simulink model "Boeing787_Yue"  (R2013a)
settings: Solver=ode23tb  SolverMode=SingleTasking  StartTime=0.0  StopTime=346  RelTol=1e-3
InitFcn:
  | load('SampleOutput.mat')
  | 
  | load('SampleFuelBurn.mat')
values from neighbouring files (symbols this model uses):
  FuelBurn = [0 0 0 0 0 0 0 0 0 0 0 0 ... (18249 elements, 1x18249)]    [Benchmark_data1.mat]
undefined symbols (not defined in the file or in its folder): ailerons, AirProp, B_737, elevator, HydProp, landing_gear, rudder, thrust_rev
libraries: PowerFlowLib x118, simulink x20
(part 18 of 26)

== system Boeing787_Yue/Electrical/Generation Unit Sync-Sync6 ==
  engine speed : Inport
  idq0 : Inport  Port=2
  Temperature : Inport  Port=3
  Bus Creator : BusCreator  Inputs=3
  Bus Creator1 : BusCreator  Inputs=3
  Coeff of Resistance : Gain  Gain=3.85e-3
  Demux : Demux  Outputs=3
  Gain : Gain  Gain=200*2/3
  Gain1 : Gain  Gain=200
  Generator : Subsystem
      mask Display:
      | p = 0:0.1:(2*pi+0.1);
      | plot(sin(p), cos(p));
      | p1 = (-pi/8-0.1-0.2):0.1:(pi/8+0.1-0.2);
      | plot(0.8*sin(p1), 0.8*cos(p1), 0.8*sin(p1+pi), 0.8*cos(p1+pi));
      | p2 = sin((-pi/8-0.1-0.2+pi/8+0.1-0.2)/2);
      | p3 = sin((-pi/8-0.1-0.2+pi/8+0.1-0.2)/2+pi);
      | p4 = cos((-pi/8-0.1-0.2+pi/8+0.1-0.2)/2);
      | p5 = cos((-pi/8-0.1-0.2+pi/8+0.1-0.2)/2+pi);
      | plot(0.8*[p2, p3], 0.8*[p4, p5]);
      | port_label('output', 1, 'Vdq0');
      | port_label('output', 2, 'Te');
      | port_label('output', 3, 'Vfd');
      | port_label('output', 4, 'Ploss');
      | port_label('input', 1, 'idq0');
      | port_label('input', 2, 'w');
      | port_label('input', 3, 'ifd');
  Initial Temperature : Constant  Value=25
  Memory : Memory
  Permanent Magnet Synchronous Generator1 : PowerFlowLib/Energy & Power Systems/Electrical/Machines/Permanent Magnet Synchronous Generator1
  RPM_to_radps : Gain  Gain=pi/30
  Scope2 : Scope
      settings: TimeRange=100  YMin=0  YMax=5500
  Sum : Sum  Inputs=++|
  Sum1 : Sum
  Sum5 : Sum  Inputs=|+-
  Sum6 : Sum  Inputs=|++
  control1 : Constant
  data_sink : PowerFlowLib/Support Functions//Tools/data_sink
  one : Constant
  three-phase active rectifier Voltage Mode : PowerFlowLib/Energy & Power Systems/Electrical/Rectifiers/three-phase  active rectifier Voltage Mode  L=1  C=1e-4
  vdq0 : Outport
  engine torque : Outport  Port=2
  Ploss : Outport  Port=3
  wires:
  [R_temp_delta] -> Generator/4(Temp)
  engine speed/1 -> RPM_to_radps/1
  Bus Creator1/1 -> Bus Creator/1  "vdq0 (V)"
  Demux/3 -> Bus Creator1/3  "v0"
  Demux/2 -> Bus Creator1/2  "vq"
  Demux/1 -> Bus Creator1/1  "vd"
  Bus Creator/1 -> data_sink/1
  Sum/1 -> engine torque/1
  RPM_to_radps/1 -> Scope2/1, Generator/2(w), Permanent Magnet Synchronous Generator1/2
  Permanent Magnet Synchronous Generator1/1 -> three-phase active rectifier Voltage Mode/1
  control1/1 -> three-phase active rectifier Voltage Mode/2
  Generator/3(vfd') -> Gain1/1
  Gain1/1 -> three-phase active rectifier Voltage Mode/3
  Gain/1 -> Generator/3(ifd'), Bus Creator/3  "Excit current (A)"
  three-phase active rectifier Voltage Mode/1 -> Gain/1
  three-phase active rectifier Voltage Mode/2 -> Memory/1
  Permanent Magnet Synchronous Generator1/2 -> Sum/1
  Generator/2(Te) -> Sum/2
  Generator/1(vdq0) -> Demux/1, vdq0/1  "Vdq0 (V)"
  Permanent Magnet Synchronous Generator1/3 -> Sum1/1
  Generator/4(Ploss) -> Sum1/2
  Sum1/1 -> Bus Creator/2, Ploss/1  "Ploss (W)"
  Memory/1 -> Permanent Magnet Synchronous Generator1/1
  Sum6/1 -> [R_temp_delta]
  one/1 -> Sum6/2
  Coeff of Resistance/1 -> Sum6/1
  Sum5/1 -> Coeff of Resistance/1
  Initial Temperature/1 -> Sum5/2
  Temperature/1 -> Sum5/1
  idq0/1 -> Generator/1(idq0)

== system Boeing787_Yue/Electrical/Loads ==
  Constant : Constant  Value=[150,0,0]
  Constant1 : Constant  Value=[150 0 0]
  Constant2 : Constant  Value=[150 0]
  Constant3 : Constant  Value=[150 0]
  ElectricalSource1 : PowerFlowLib/Support Functions//Tools/ElectricalSource  Tag=Flow  Description=TwoPhase  load_loc=Cockpit  ACDC_load=DC
      link override From1: GotoTag=RightWing_ElecAC_9219
      link override From2: GotoTag=RightWing_ElecAC_5921
  ElectricalSource4 : PowerFlowLib/Support Functions//Tools/ElectricalSource  Tag=Flow  Description=TwoPhase  load_loc=RightWing  ACDC_load=AC
      link override From1: GotoTag=RightWing_ElecAC_9219
      link override From2: GotoTag=RightWing_ElecAC_5921
  ElectricalSource5 : PowerFlowLib/Support Functions//Tools/ElectricalSource  Tag=Flow  Description=TwoPhase  load_loc=RightWing  ACDC_load=AC
      link override From1: GotoTag=RightWing_ElecAC_9219
      link override From2: GotoTag=RightWing_ElecAC_5921
  ElectricalSource6 : PowerFlowLib/Support Functions//Tools/ElectricalSource  Tag=Flow  Description=TwoPhase  load_loc=Cabin  ACDC_load=DC
      link override From1: GotoTag=RightWing_ElecAC_9219
      link override From2: GotoTag=RightWing_ElecAC_5921
  Reactive Power : Gain  Gain=[0 1 0]
  Reactive Power1 : Gain  Gain=[0 1 0]
  "Real Power " : Gain  Gain=[0 1]
  "Real Power  " : Gain  Gain=[1 0 0]
  Real Power  1 : Gain  Gain=[1 0 0]
  Real Power 1 : Gain  Gain=[0 1]
  Scope{,1..7} (8 alike) : Scope
      Scope settings: YMin=-10  YMax=10  SaveName=ScopeData14
      Scope1 settings: YMin=-10  YMax=10  SaveName=ScopeData15
      Scope2 settings: YMin=101.20265  YMax=191.19996  SaveName=ScopeData16
      Scope3 settings: YMin=-1.00000  YMax=1.00000  SaveName=ScopeData17
      Scope4 settings: YMin=-3473949.375  YMax=385994.375  SaveName=ScopeData18
      Scope5 settings: YMin=-280526.36068  YMax=201966.60807  SaveName=ScopeData19
      Scope6 settings: ShowLegends=on  YMin=-1.00000  YMax=1.00000  SaveName=ScopeData20
      Scope7 settings: YMin=-1.00000  YMax=1.00000  SaveName=ScopeData22
  Sum : Sum  Inputs=|++
  Sum of Elements{,1..3} (4 alike) : Sum  Inputs=+
  Sum1 : Sum  Inputs=|++
  230 Vac Loads : Outport
  115 Vac Loads : Outport  Port=2
  270 Vdc Loads : Outport  Port=3
  28 Vdc Loads : Outport  Port=4
  wires:
  "Real Power  "/1 -> Sum/1
  Reactive Power/1 -> Sum/2
  Sum of Elements/1 -> "Real Power  "/1
  Sum of Elements1/1 -> Reactive Power/1
  Sum/1 -> Scope4/1
  Real Power  1/1 -> Sum1/1
  Reactive Power1/1 -> Sum1/2
  Sum of Elements2/1 -> Real Power  1/1
  Sum of Elements3/1 -> Reactive Power1/1
  Sum1/1 -> Scope5/1
  "Real Power "/1 -> Scope6/1
  ElectricalSource6/1 -> Scope2/1, "Real Power "/1
  Real Power 1/1 -> Scope7/1
  ElectricalSource5/1 -> Scope/1, Sum of Elements/1
  ElectricalSource4/1 -> Scope1/1, Sum of Elements2/1
  ElectricalSource1/1 -> Scope3/1, Real Power 1/1
  Constant/1 -> 230 Vac Loads/1
  Constant1/1 -> 115 Vac Loads/1
  Constant2/1 -> 270 Vdc Loads/1
  Constant3/1 -> 28 Vdc Loads/1

== system Boeing787_Yue/Electrical/Outputs ==
  Left_Wing_Toqrue_Nm : Inport
  Rght_Wing_Torque_Nm : Inport  Port=2
  APU_Torque_Nm : Inport  Port=3
  DC_Voltage_270 : Inport  Port=4
  Bus Creator : BusCreator
  Electrical : Outport
  wires:
  Rght_Wing_Torque_Nm/1 -> Bus Creator/2  "Right Wing Torq (Nm)"
  APU_Torque_Nm/1 -> Bus Creator/3  "APU Torq (Nm)"
  Left_Wing_Toqrue_Nm/1 -> Bus Creator/1  "Left Wing Torq (Nm)"
  Bus Creator/1 -> Electrical/1
  DC_Voltage_270/1 -> Bus Creator/4  "DC_Voltage_270"

== system Boeing787_Yue/Electrical/Thermal Interface ==
  Left_Wing_SCVGU_Ploss_W : Inport
  Right_Wing_SCVGU_Ploss_W : Inport  Port=2
  APU_Ploss_W : Inport  Port=3
  Inverter_Ploss_W : Inport  Port=4
  Battery1_Ploss_W : Inport  Port=5
  Battery2_Ploss_W : Inport  Port=6
  Backup_Battery_Ploss_W : Inport  Port=7
  Loadloss_W : Inport  Port=8
  Mux : Mux
  Sum : Sum
  Terminator{,1..3} (4 alike) : Terminator
  ThermalSink : PowerFlowLib/Support Functions//Tools/ThermalSink  Tag=Flow  Description=TwoPhase  load_loc=Cabin  units=Watts  unq_id=8332
  To Workspace : ToWorkspace  VariableName=Tot_Gen_Loss_W  SampleTime=10  SaveFormat=Structure With Time
  wires:
  Right_Wing_SCVGU_Ploss_W/1 -> Sum/2, Terminator1/1
  APU_Ploss_W/1 -> Terminator2/1
  Mux/1 -> ThermalSink/1
  Inverter_Ploss_W/1 -> Mux/1
  Battery1_Ploss_W/1 -> Mux/2
  Battery2_Ploss_W/1 -> Mux/3
  Backup_Battery_Ploss_W/1 -> Mux/4
  Loadloss_W/1 -> Terminator3/1
  Left_Wing_SCVGU_Ploss_W/1 -> Sum/1, Terminator/1
  Sum/1 -> To Workspace/1

== system Boeing787_Yue/Eng1/Gearbox ==
  w_engine : Inport
  T_gen : Inport  Port=2
  1-tran_efficiency : Gain  Gain=1-Gear_Efficiency/100  SaturateOnIntegerOverflow=on  OutDataTypeStr=Inherit: Same as input  ParamDataTypeStr=Inherit: Same as input
  Gain : Gain  Gain=Gear_Ratio
  Gain1 : Gain  Gain=Gear_Ratio
  Memory1 : Memory
  Sum : Sum  Inputs=-++  SaturateOnIntegerOverflow=on  InputSameDT=on  OutDataTypeStr=Inherit: Same as first input
  gear1 NL loss : Lookup  InputValues=[0;1000;2000;3000;4000;5000;6000]*2*pi/60  Table=[0;0.735;1.334;1.491;1.525;1.212;1.276]  SaturateOnIntegerOverflow=on
  tran_efficiency : Gain  Gain=Gear_Efficiency/4/100  SaturateOnIntegerOverflow=on  OutDataTypeStr=Inherit: Same as input  ParamDataTypeStr=Inherit: Same as input
  w_shaft : Outport
  T_shaft : Outport  Port=2
  wires:
  Gain/1 -> w_shaft/1
  Gain1/1 -> Memory1/1
  T_gen/1 -> Gain1/1, 1-tran_efficiency/1
  w_engine/1 -> Gain/1, gear1 NL loss/1
  gear1 NL loss/1 -> tran_efficiency/1
  Memory1/1 -> Sum/3
  1-tran_efficiency/1 -> Sum/2
  tran_efficiency/1 -> Sum/1
  Sum/1 -> T_shaft/1

== system Boeing787_Yue/Eng1/Unit Conversion  ==
  Signal_in : Inport
  conv_fcn : Fcn  Expr=u(1)/745.69987
  Converted Signal Out : Outport
  wires:
  Signal_in/1 -> conv_fcn/1
  conv_fcn/1 -> Converted Signal Out/1

== system Boeing787_Yue/Eng1/Unit Conversion 1 ==
  Signal_in : Inport
  conv_fcn : Fcn  Expr=u(1)/1.8
  Converted Signal Out : Outport
  wires:
  conv_fcn/1 -> Converted Signal Out/1
  Signal_in/1 -> conv_fcn/1

== system Boeing787_Yue/Eng1/Unit Conversion 2 ==
  Signal_in : Inport
  conv_fcn : Fcn  Expr=u(1)/.45359237
  Converted Signal Out : Outport
  wires:
  conv_fcn/1 -> Converted Signal Out/1
  Signal_in/1 -> conv_fcn/1

== system Boeing787_Yue/Eng1/Unit Conversion 3 ==
  Signal_in : Inport
  conv_fcn : Fcn  Expr=u(1)/.45359237
  Converted Signal Out : Outport
  wires:
  conv_fcn/1 -> Converted Signal Out/1
  Signal_in/1 -> conv_fcn/1

== system Boeing787_Yue/Eng1/Unit Conversion 4 ==
  Signal_in : Inport
  conv_fcn : Fcn  Expr=u(1)/(1.450377e-1)
  Converted Signal Out : Outport
  wires:
  Signal_in/1 -> conv_fcn/1
  conv_fcn/1 -> Converted Signal Out/1

== system Boeing787_Yue/Eng1/Unit Conversion 5 ==
  Signal_in : Inport
  conv_fcn : Fcn  Expr=u(1)*.45359237
  Converted Signal Out : Outport
  wires:
  Signal_in/1 -> conv_fcn/1
  conv_fcn/1 -> Converted Signal Out/1

== system Boeing787_Yue/Eng2/Gearbox ==
  w_engine : Inport
  T_gen : Inport  Port=2
  1-tran_efficiency : Gain  Gain=1-Gear_Efficiency/100  SaturateOnIntegerOverflow=on  OutDataTypeStr=Inherit: Same as input  ParamDataTypeStr=Inherit: Same as input
  Gain : Gain  Gain=Gear_Ratio
  Gain1 : Gain  Gain=Gear_Ratio
  Memory1 : Memory
  Sum : Sum  Inputs=-++  SaturateOnIntegerOverflow=on  InputSameDT=on  OutDataTypeStr=Inherit: Same as first input
  gear1 NL loss : Lookup  InputValues=[0;1000;2000;3000;4000;5000;6000]*2*pi/60  Table=[0;0.735;1.334;1.491;1.525;1.212;1.276]  SaturateOnIntegerOverflow=on
  tran_efficiency : Gain  Gain=Gear_Efficiency/4/100  SaturateOnIntegerOverflow=on  OutDataTypeStr=Inherit: Same as input  ParamDataTypeStr=Inherit: Same as input
  w_shaft : Outport
  T_shaft : Outport  Port=2
  wires:
  Sum/1 -> T_shaft/1
  tran_efficiency/1 -> Sum/1
  1-tran_efficiency/1 -> Sum/2
  Memory1/1 -> Sum/3
  gear1 NL loss/1 -> tran_efficiency/1
  w_engine/1 -> gear1 NL loss/1, Gain/1
  T_gen/1 -> 1-tran_efficiency/1, Gain1/1
  Gain1/1 -> Memory1/1
  Gain/1 -> w_shaft/1

== system Boeing787_Yue/Eng2/Unit Conversion  ==
  Signal_in : Inport
  conv_fcn : Fcn  Expr=u(1)/745.69987
  Converted Signal Out : Outport
  wires:
  conv_fcn/1 -> Converted Signal Out/1
  Signal_in/1 -> conv_fcn/1

== system Boeing787_Yue/Eng2/Unit Conversion 1 ==
  Signal_in : Inport
  conv_fcn : Fcn  Expr=u(1)/1.8
  Converted Signal Out : Outport
  wires:
  Signal_in/1 -> conv_fcn/1
  conv_fcn/1 -> Converted Signal Out/1

== system Boeing787_Yue/Eng2/Unit Conversion 2 ==
  Signal_in : Inport
  conv_fcn : Fcn  Expr=u(1)/.45359237
  Converted Signal Out : Outport
  wires:
  Signal_in/1 -> conv_fcn/1
  conv_fcn/1 -> Converted Signal Out/1

== system Boeing787_Yue/Eng2/Unit Conversion 3 ==
  Signal_in : Inport
  conv_fcn : Fcn  Expr=u(1)/.45359237
  Converted Signal Out : Outport
  wires:
  Signal_in/1 -> conv_fcn/1
  conv_fcn/1 -> Converted Signal Out/1

== system Boeing787_Yue/Eng2/Unit Conversion 4 ==
  Signal_in : Inport
  conv_fcn : Fcn  Expr=u(1)/(1.450377e-1)
  Converted Signal Out : Outport
  wires:
  conv_fcn/1 -> Converted Signal Out/1
  Signal_in/1 -> conv_fcn/1

== system Boeing787_Yue/Eng2/Unit Conversion 5 ==
  Signal_in : Inport
  conv_fcn : Fcn  Expr=u(1)*.45359237
  Converted Signal Out : Outport
  wires:
  conv_fcn/1 -> Converted Signal Out/1
  Signal_in/1 -> conv_fcn/1

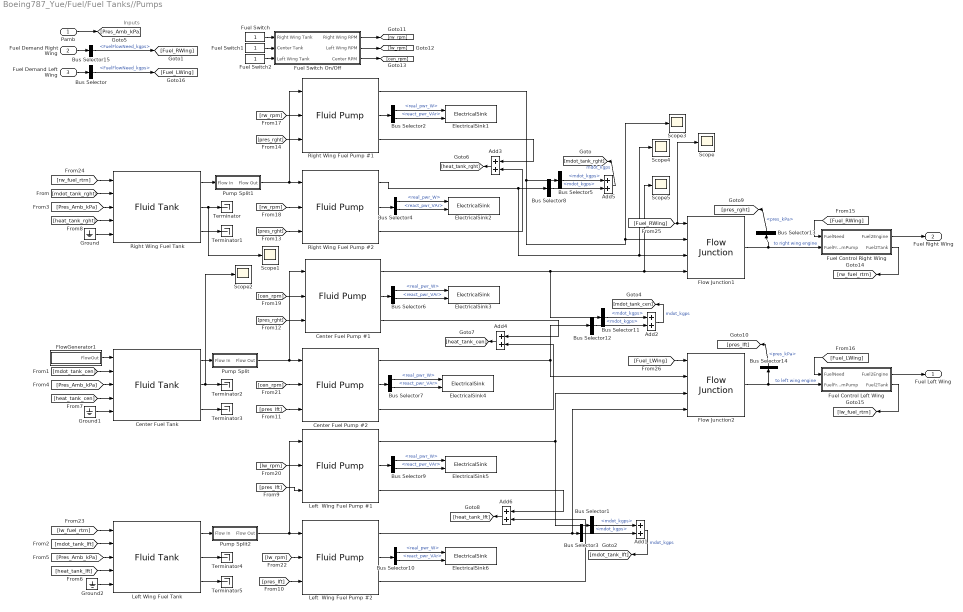
== system Boeing787_Yue/Fuel/Fuel Tanks//Pumps ==
  note: Inputs
  Pamb : Inport
  Fuel Demand Right Wing : Inport  Port=2
  Fuel Demand Left Wing : Inport  Port=3
  Add{1..6} (6 alike) : Sum
  Bus Selector : BusSelector  OutputSignals=Fuel.FuelFlowNeed_kgps
  Bus Selector{1,3,5,8,11..12} (6 alike) : BusSelector  OutputSignals=mdot_kgps
  Bus Selector{2,4,6..7,9..10} (6 alike) : BusSelector  OutputSignals=real_pwr_W,react_pwr_VAr
  Bus Selector13 : BusSelector  OutputSignals=pres_kPa
  Bus Selector14 : BusSelector  OutputSignals=pres_kPa
  Bus Selector15 : BusSelector  OutputSignals=Fuel.FuelFlowNeed_kgps
  Center Fuel Pump #1 : PowerFlowLib/Energy & Power Systems/Thermal/Fuel & Oil/Fluid Pump  fld=Fuel  maptype=Pressure (kPa) vs. Vol. Flow Rate (m³/hr)  map=B737_AC_fuel1  map_load=off  SG=0.82  pump_eff=.75  heat_out=off  AC_pwr=on  pf=1  mech_pwr=off
  Center Fuel Pump #2 : PowerFlowLib/Energy & Power Systems/Thermal/Fuel & Oil/Fluid Pump  fld=Fuel  maptype=Pressure (kPa) vs. Vol. Flow Rate (m³/hr)  map=B737_AC_fuel1  map_load=off  SG=0.82  pump_eff=.75  heat_out=off  AC_pwr=on  pf=1  mech_pwr=off
  Center Fuel Tank : PowerFlowLib/Energy & Power Systems/Thermal/Fuel & Oil/Fluid Tank  fld=Fuel  fileslct=off  filename=fueltank_area.m  filedir=fueltank_area.m  tank_loc=Left Wing Tank  areaprompt2=off  max_vol=3.2  m_init=2500  fld_Tint=0  ull_Tint=30  Pover=100  HTC_fg=14.2  wallHXF=off  wetHTC=14.2  dryHTC=14.2  Qinternal=0
  ElectricalSink1 : PowerFlowLib/Support Functions//Tools/ElectricalSink  Tag=Flow  Description=TwoPhase  load_loc=RightWing  ACDC_load=AC  units=Watts  unq_id=1878
  ElectricalSink2 : PowerFlowLib/Support Functions//Tools/ElectricalSink  Tag=Flow  Description=TwoPhase  load_loc=RightWing  ACDC_load=AC  units=Watts  unq_id=3506
  ElectricalSink3 : PowerFlowLib/Support Functions//Tools/ElectricalSink  Tag=Flow  Description=TwoPhase  load_loc=RightWing  ACDC_load=AC  units=Watts  unq_id=5921
  ElectricalSink4 : PowerFlowLib/Support Functions//Tools/ElectricalSink  Tag=Flow  Description=TwoPhase  load_loc=LeftWing  ACDC_load=AC  units=Watts  unq_id=9617
  ElectricalSink5 : PowerFlowLib/Support Functions//Tools/ElectricalSink  Tag=Flow  Description=TwoPhase  load_loc=LeftWing  ACDC_load=AC  units=Watts  unq_id=9683
  ElectricalSink6 : PowerFlowLib/Support Functions//Tools/ElectricalSink  Tag=Flow  Description=TwoPhase  load_loc=LeftWing  ACDC_load=AC  units=Watts  unq_id=2418
  Flow Junction1 : PowerFlowLib/Energy & Power Systems/Thermal/Fuel & Oil/Flow Junction  Description=TwoPhase  fld=Fuel  V=.05  Bm=10^5  initPres=6000  initTemp=30
  Flow Junction2 : PowerFlowLib/Energy & Power Systems/Thermal/Fuel & Oil/Flow Junction  Description=TwoPhase  fld=Fuel  V=.05  Bm=10^5  initPres=6000  initTemp=30
  FlowGenerator1 : Subsystem  Tag=Flow  Description=TwoPhase  mask{fld_type1=null, flowrate=0, flowtemp=0, flowpres=00, flowenthalpy=0}
      mask prompts: fld_type1 "Fluid Type"; flowrate "Fluid Flow Rate (kg/s)"; flowtemp "Fluid Flow Temperature (C)"; flowpres "Fluid Flow Pressure (kPa)"; flowenthalpy "Fluid Flow Enthalpy (kJ/kg)"
      mask TypeOptions fld_type1: null
      mask Display: text(.5,.5,'Flow Source','horizontalAlignment','center','texmode','on')
  Fuel Control Left Wing : Subsystem
      mask Display:
      | port_label('input',1,'{\bf Fuel Need}','TexMode','on')
      | port_label('input',2,'{\bf Fuel In}','TexMode','on')
      | 
      | 
      | port_label('output',1,'{\bf Fuel to Eng.}','TexMode','on')
      | port_label('output',2,'{\bf Fuel Return}','TexMode','on')
  "Fuel Control Right Wing " : Subsystem
      mask Display:
      | port_label('input',1,'{\bf Fuel Need}','TexMode','on')
      | port_label('input',2,'{\bf Fuel In}','TexMode','on')
      | 
      | 
      | port_label('output',1,'{\bf Fuel to Eng.}','TexMode','on')
      | port_label('output',2,'{\bf Fuel Return}','TexMode','on')
  Fuel Switch : Constant
  Fuel Switch On/Off : Subsystem
  Fuel Switch1 : Constant
  Fuel Switch2 : Constant
  Ground : Ground
  Ground1 : Ground
  Ground2 : Ground
  Left  Wing Fuel Pump #1 : PowerFlowLib/Energy & Power Systems/Thermal/Fuel & Oil/Fluid Pump  fld=Fuel  maptype=Pressure (kPa) vs. Vol. Flow Rate (m³/hr)  map=B737_AC_fuel1  map_load=off  SG=0.82  pump_eff=.75  heat_out=off  AC_pwr=on  pf=1  mech_pwr=off
  Left  Wing Fuel Pump #2 : PowerFlowLib/Energy & Power Systems/Thermal/Fuel & Oil/Fluid Pump  fld=Fuel  maptype=Pressure (kPa) vs. Vol. Flow Rate (m³/hr)  map=B737_AC_fuel1  map_load=off  SG=0.82  pump_eff=.75  heat_out=off  AC_pwr=on  pf=1  mech_pwr=off
  Left Wing Fuel Tank : PowerFlowLib/Energy & Power Systems/Thermal/Fuel & Oil/Fluid Tank  fld=Fuel  fileslct=off  filename=fueltank_area.m  filedir=fueltank_area.m  tank_loc=Left Wing Tank  areaprompt2=off  max_vol=3.2  m_init=2500  fld_Tint=0  ull_Tint=30  Pover=100  HTC_fg=14.2  wallHXF=off  wetHTC=14.2  dryHTC=14.2  Qinternal=0
  Pump Split : Subsystem
  Pump Split1 : Subsystem
  Pump Split2 : Subsystem
  Right Wing Fuel Pump #1 : PowerFlowLib/Energy & Power Systems/Thermal/Fuel & Oil/Fluid Pump  fld=Fuel  maptype=Pressure (kPa) vs. Vol. Flow Rate (m³/hr)  map=B737_AC_fuel1  map_load=off  SG=0.82  pump_eff=.75  heat_out=off  AC_pwr=on  pf=1  mech_pwr=off
  Right Wing Fuel Pump #2 : PowerFlowLib/Energy & Power Systems/Thermal/Fuel & Oil/Fluid Pump  fld=Fuel  maptype=Pressure (kPa) vs. Vol. Flow Rate (m³/hr)  map=B737_AC_fuel1  map_load=off  SG=0.82  pump_eff=.75  heat_out=off  AC_pwr=on  pf=1  mech_pwr=off
  Right Wing Fuel Tank : PowerFlowLib/Energy & Power Systems/Thermal/Fuel & Oil/Fluid Tank  fld=Fuel  fileslct=off  filename=fueltank_area.m  filedir=fueltank_area.m  tank_loc=Left Wing Tank  areaprompt2=off  max_vol=3.2  m_init=2500  fld_Tint=0  ull_Tint=30  Pover=100  HTC_fg=14.2  wallHXF=off  wetHTC=14.2  dryHTC=14.2  Qinternal=0
  Scope{,1..5} (6 alike) : Scope
      Scope settings: SaveName=ScopeData21
      Scope1 settings: YMin=2498.9  YMax=2498.9  SaveName=ScopeData23
      Scope2 settings: SaveName=ScopeData25
      Scope3 settings: YMin=-500  YMax=500  SaveName=ScopeData27
      Scope4 settings: YMin=-500  YMax=500  SaveName=ScopeData28
      Scope5 settings: SaveName=ScopeData29
  Terminator{,1..5} (6 alike) : Terminator
  Fuel Left Wing : Outport
  Fuel Right Wing : Outport  Port=2
  wires:
  Pamb/1 -> [Pres_Amb_kPa]
  Fuel Switch/1 -> Fuel Switch On/Off/1(Right Wing Tank)
  Fuel Switch1/1 -> Fuel Switch On/Off/2(Center Tank)
  Fuel Switch2/1 -> Fuel Switch On/Off/3(Left Wing Tank)
  Fuel Switch On/Off/1(Right Wing RPM) -> [rw_rpm]
  Fuel Switch On/Off/2(Left Wing RPM) -> [lw_rpm]
  Fuel Switch On/Off/3(Center RPM) -> [cen_rpm]
  Left  Wing Fuel Pump #2/1 -> Flow Junction2/4, Bus Selector3/1
  [lw_fuel_rtrn] -> Left Wing Fuel Tank/1
  Left  Wing Fuel Pump #2/2 -> Bus Selector10/1
  Left  Wing Fuel Pump #1/1 -> Flow Junction2/3, Bus Selector1/1
  Left  Wing Fuel Pump #1/2 -> Bus Selector9/1
  Center Fuel Pump #2/1 -> Flow Junction2/2, Bus Selector12/1
  FlowGenerator1/1(FlowOut) -> Center Fuel Tank/1
  Center Fuel Pump #2/2 -> Bus Selector7/1
  Flow Junction2/1 -> Bus Selector14/1, Fuel Control Left Wing/2(FuelFromPump)  "to left wing engine"
  Center Fuel Pump #1/1 -> Bus Selector11/1, Flow Junction1/4, Scope5/1
  Center Fuel Pump #1/2 -> Bus Selector6/1
  Flow Junction1/1 -> Bus Selector13/1, "Fuel Control Right Wing "/2(FuelFromPump)  "to right wing engine"
  Center Fuel Tank/1 -> Pump Split/1(Flow In)
  Right Wing Fuel Pump #2/1 -> Bus Selector8/1, Flow Junction1/3, Scope4/1
  [rw_fuel_rtrn] -> Right Wing Fuel Tank/1
  Right Wing Fuel Pump #2/2 -> Bus Selector4/1
  Right Wing Fuel Pump #1/1 -> Bus Selector5/1, Flow Junction1/2, Scope3/1
  [rw_rpm] -> Right Wing Fuel Pump #1/2
  Right Wing Fuel Tank/1 -> Pump Split1/1(Flow In)
  Pump Split1/1(Flow Out) -> Right Wing Fuel Pump #2/1, Right Wing Fuel Pump #1/1
  Bus Selector8/1 -> Add5/2  "<mdot_kgps>"
  [mdot_tank_rght] -> Right Wing Fuel Tank/2
  [mdot_tank_cen] -> Center Fuel Tank/2
  [mdot_tank_lft] -> Left Wing Fuel Tank/2
  Pump Split/1(Flow Out) -> Center Fuel Pump #1/1, Center Fuel Pump #2/1
  Left Wing Fuel Tank/1 -> Pump Split2/1(Flow In)
  Bus Selector5/1 -> Add5/1  "<mdot_kgps>"
  Add5/1 -> [mdot_tank_rght]  "mdot_kgps"
  Bus Selector3/1 -> Add1/2  "<mdot_kgps>"
  Bus Selector1/1 -> Add1/1  "<mdot_kgps>"
  Add1/1 -> [mdot_tank_lft]  "mdot_kgps"
  Bus Selector12/1 -> Add2/2  "<mdot_kgps>"
  Bus Selector11/1 -> Add2/1  "<mdot_kgps>"
  Add2/1 -> [mdot_tank_cen]  "mdot_kgps"
  [Pres_Amb_kPa] -> Right Wing Fuel Tank/3
  [Pres_Amb_kPa] -> Center Fuel Tank/3
  [Pres_Amb_kPa] -> Left Wing Fuel Tank/3
  Add6/1 -> [heat_tank_lft]
  [heat_tank_lft] -> Left Wing Fuel Tank/4
  [heat_tank_cen] -> Center Fuel Tank/4
  [heat_tank_rght] -> Right Wing Fuel Tank/4
  Bus Selector13/1 -> [pres_rght]  "<pres_kPa>"
  [rw_rpm] -> Right Wing Fuel Pump #2/2
  [cen_rpm] -> Center Fuel Pump #1/2
  [cen_rpm] -> Center Fuel Pump #2/2
  [lw_rpm] -> Left  Wing Fuel Pump #1/2
  [lw_rpm] -> Left  Wing Fuel Pump #2/2
  Bus Selector14/1 -> [pres_lft]  "<pres_kPa>"
  [pres_lft] -> Left  Wing Fuel Pump #1/3
  [pres_lft] -> Left  Wing Fuel Pump #2/3
  [pres_lft] -> Center Fuel Pump #2/3
  [pres_rght] -> Center Fuel Pump #1/3
  [pres_rght] -> Right Wing Fuel Pump #2/3
  [pres_rght] -> Right Wing Fuel Pump #1/3
  [Fuel_LWing] -> Flow Junction2/1
  [Fuel_RWing] -> Flow Junction1/1, Scope/1
  Right Wing Fuel Tank/2 -> Terminator/1, Scope1/1
  Right Wing Fuel Tank/3 -> Terminator1/1
  Center Fuel Tank/2 -> Terminator2/1, Scope2/1
  Center Fuel Tank/3 -> Terminator3/1
  Left Wing Fuel Tank/2 -> Terminator4/1
  Left Wing Fuel Tank/3 -> Terminator5/1
  Ground/1 -> Right Wing Fuel Tank/5
  Ground1/1 -> Center Fuel Tank/5
  Ground2/1 -> Left Wing Fuel Tank/5
  Fuel Demand Left Wing/1 -> Bus Selector/1
  [Fuel_RWing] -> "Fuel Control Right Wing "/1(FuelNeed)
  [Fuel_LWing] -> Fuel Control Left Wing/1(FuelNeed)
  Fuel Control Left Wing/2(Fuel2Tank) -> [lw_fuel_rtrn]
  "Fuel Control Right Wing "/2(Fuel2Tank) -> [rw_fuel_rtrn]
  "Fuel Control Right Wing "/1(Fuel2Engine) -> Fuel Right Wing/1
  Fuel Control Left Wing/1(Fuel2Engine) -> Fuel Left Wing/1
  Pump Split2/1(Flow Out) -> Left  Wing Fuel Pump #1/1, Left  Wing Fuel Pump #2/1
  Bus Selector/1 -> [Fuel_LWing]  "<FuelFlowNeed_kgps>"
  Fuel Demand Right Wing/1 -> Bus Selector15/1
  Bus Selector15/1 -> [Fuel_RWing]  "<FuelFlowNeed_kgps>"
  Bus Selector2/1 -> ElectricalSink1/1  "<real_pwr_W>"
  Add4/1 -> [heat_tank_cen]
  Add3/1 -> [heat_tank_rght]
  Right Wing Fuel Pump #1/2 -> Bus Selector2/1
  Bus Selector2/2 -> ElectricalSink1/2  "<react_pwr_VAr>"
  Bus Selector4/1 -> ElectricalSink2/1  "<real_pwr_W>"
  Bus Selector4/2 -> ElectricalSink2/2  "<react_pwr_VAr>"
  Bus Selector6/1 -> ElectricalSink3/1  "<real_pwr_W>"
  Bus Selector6/2 -> ElectricalSink3/2  "<react_pwr_VAr>"
  Bus Selector7/1 -> ElectricalSink4/1  "<real_pwr_W>"
  Bus Selector7/2 -> ElectricalSink4/2  "<react_pwr_VAr>"
  Bus Selector9/1 -> ElectricalSink5/1  "<real_pwr_W>"
  Bus Selector9/2 -> ElectricalSink5/2  "<react_pwr_VAr>"
  Bus Selector10/1 -> ElectricalSink6/1  "<real_pwr_W>"
  Bus Selector10/2 -> ElectricalSink6/2  "<react_pwr_VAr>"
  Right Wing Fuel Pump #1/3 -> Add3/1
  Right Wing Fuel Pump #2/3 -> Add3/2
  Center Fuel Pump #1/3 -> Add4/1
  Center Fuel Pump #2/3 -> Add4/2
  Left  Wing Fuel Pump #1/3 -> Add6/1
  Left  Wing Fuel Pump #2/3 -> Add6/2

== system Boeing787_Yue/Fuel/Oil Tanks//Pumps Left Wing ==
  Oil Sys Pres : Inport
  Flow In : Inport  Port=2
  Bus Selector1 : BusSelector  OutputSignals=Oil
  Bus Selector2 : BusSelector  OutputSignals=real_pwr_W,react_pwr_VAr
  Bus Selector5 : BusSelector  OutputSignals=mdot_kgps,pres_kPa
  ElectricalSink1 : PowerFlowLib/Support Functions//Tools/ElectricalSink  Tag=Flow  Description=TwoPhase  load_loc=LeftWing  ACDC_load=AC  units=Watts  unq_id=9734
  Fluid Pump : PowerFlowLib/Energy & Power Systems/Thermal/Fuel & Oil/Fluid Pump  fld=Fuel  maptype=Pressure (kPa) vs. Vol. Flow Rate (m³/hr)  map=B737_AC_oil1  map_load=off  SG=0.82  pump_eff=.75  heat_out=off  AC_pwr=on  pf=1  mech_pwr=off
  Fluid Tank : PowerFlowLib/Energy & Power Systems/Thermal/Fuel & Oil/Fluid Tank  fld=Fuel  fileslct=off  filename=oiltank_area.m  filedir=C:\Users\mwillms4\Documents\GitHub\PowerFlow\SupportFunctions\oiltank_area.m  tank_loc=Left Wing Tank  areaprompt2=off  max_vol=0.00757082  m_init=5.5  fld_Tint=20  ull_Tint=30  Pover=100  HTC_fg=14.2  wallHXF=off  wetHTC=14.2  dryHTC=14.2  Qinternal=0
  Fuel Switch2 : Constant  Value=1400
  Ground : Ground
  Ground1 : Ground
  Terminator : Terminator
  Terminator1 : Terminator
  Oil To HX : Outport
  wires:
  Bus Selector5/1 -> Fluid Tank/2  "<mdot_kgps>"
  Fuel Switch2/1 -> Fluid Pump/2
  Flow In/1 -> Bus Selector1/1
  Oil Sys Pres/1 -> Fluid Pump/3
  Ground1/1 -> Fluid Tank/3
  Fluid Pump/1 -> Oil To HX/1, Bus Selector5/1
  Fluid Pump/3 -> Fluid Tank/4
  Ground/1 -> Fluid Tank/5
  Fluid Tank/3 -> Terminator1/1
  Fluid Tank/2 -> Terminator/1
  Fluid Tank/1 -> Fluid Pump/1
  Bus Selector2/1 -> ElectricalSink1/1  "<real_pwr_W>"
  Bus Selector2/2 -> ElectricalSink1/2  "<react_pwr_VAr>"
  Fluid Pump/2 -> Bus Selector2/1
  Bus Selector1/1 -> Fluid Tank/1  "<Oil>"

== system Boeing787_Yue/Fuel/Oil Tanks//Pumps Right Wing ==
  Oil Sys Pres : Inport
  Flow In : Inport  Port=2
  Bus Selector1 : BusSelector  OutputSignals=Oil
  Bus Selector2 : BusSelector  OutputSignals=real_pwr_W,react_pwr_VAr
  Bus Selector5 : BusSelector  OutputSignals=mdot_kgps,pres_kPa
  ElectricalSink1 : PowerFlowLib/Support Functions//Tools/ElectricalSink  Tag=Flow  Description=TwoPhase  load_loc=LeftWing  ACDC_load=AC  units=Watts  unq_id=8332
  Fluid Pump : PowerFlowLib/Energy & Power Systems/Thermal/Fuel & Oil/Fluid Pump  fld=Fuel  maptype=Pressure (kPa) vs. Vol. Flow Rate (m³/hr)  map=B737_AC_oil1  map_load=off  SG=0.82  pump_eff=.75  heat_out=off  AC_pwr=on  pf=1  mech_pwr=off
  Fluid Tank : PowerFlowLib/Energy & Power Systems/Thermal/Fuel & Oil/Fluid Tank  fld=Fuel  fileslct=off  filename=oiltank_area.m  filedir=C:\Users\mwillms4\Documents\GitHub\PowerFlow\SupportFunctions\oiltank_area.m  tank_loc=Left Wing Tank  areaprompt2=off  max_vol=0.00757082  m_init=5.5  fld_Tint=20  ull_Tint=30  Pover=100  HTC_fg=14.2  wallHXF=off  wetHTC=14.2  dryHTC=14.2  Qinternal=0
  Fuel Switch2 : Constant  Value=1400
  Ground : Ground
  Ground1 : Ground
  Terminator : Terminator
  Terminator1 : Terminator
  Oil To HX : Outport
  wires:
  Bus Selector1/1 -> Fluid Tank/1  "<Oil>"
  Fluid Pump/2 -> Bus Selector2/1
  Bus Selector2/2 -> ElectricalSink1/2  "<react_pwr_VAr>"
  Bus Selector2/1 -> ElectricalSink1/1  "<real_pwr_W>"
  Fluid Tank/1 -> Fluid Pump/1
  Fluid Tank/2 -> Terminator/1
  Fluid Tank/3 -> Terminator1/1
  Ground/1 -> Fluid Tank/5
  Fluid Pump/3 -> Fluid Tank/4
  Fluid Pump/1 -> Bus Selector5/1, Oil To HX/1
  Ground1/1 -> Fluid Tank/3
  Oil Sys Pres/1 -> Fluid Pump/3
  Flow In/1 -> Bus Selector1/1
  Fuel Switch2/1 -> Fluid Pump/2
  Bus Selector5/1 -> Fluid Tank/2  "<mdot_kgps>"

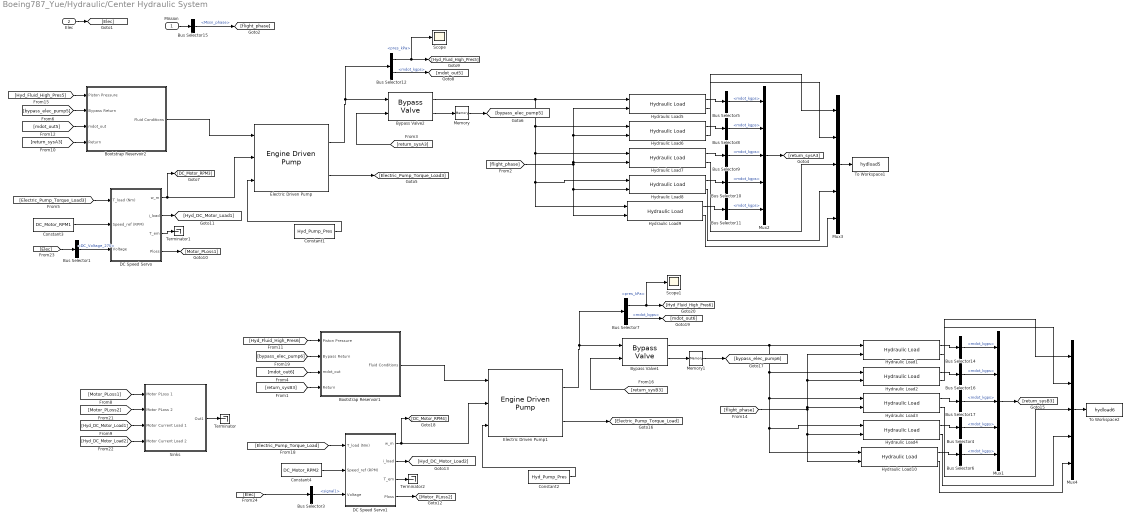
== system Boeing787_Yue/Hydraulic/Center Hydraulic System ==
  Mission : Inport
  Elec : Inport  Port=2
  Bootstrap Reservoir1 : Subsystem  mask(Fluid Reservoir){res_vol=.25, High_Pres_Area=.05, Low_Pres_Area=0, pres_loss=1, T_init=300, P_init=1500, mass_init=30}
      mask prompts: res_vol "Resevoir Volume [m³]"; High_Pres_Area "High Pressure Piston Area"; Low_Pres_Area "Low Pressure Piston Area"; pres_loss "Air Pressure Losses [%]"; T_init "Initial Fluid Temp [K]"; P_init "Initial Air Pressure [kPa]"; mass_init "Initial Fluid Mass [kg]"
      mask help:
      | The fluid reservoir serves as a tank for storing excess hydraulic fluid.
      | The reservoir is fed by returning hydraulic fluid and feeds the engine driven pump.
      | Currently the fluid reservoir tracks the time dependent mass and temperature of the hydraulic fluid in the tank.
      |
      | Block Inputs
      | #1: Bleed air properties (Bus signal)
      | #2: Bypass return from bypass valve
      | #3: Mass flow rate pumped out by hydraulic pump
      | #4: Mass flow rate returned from actuators
      |
      | Block Outputs
      | #1: Bleed air demanded to maintain pressurization
      | #2: Hydraulic fluid properties in the reservoir
      mask init:
      | load AirProp
      | load HydProp
      mask Help: eval('open(''FluidReservoir_help.html'')');
      mask Display:
      | image(imread('hyd_res.png'))
      | 
      | port_label('input',1,'{\bf High Piston Pressure}','TexMode','on')
      | port_label('input',2,'{\bf Bypass Return}','TexMode','on')
      | port_label('input',3,'{\bf m_d_o_t Out}','TexMode','on')
      | port_label('input',4,'{\bf m_d_o_t Return}','TexMode','on')
      | 
      | 
      | port_label('output',1,'{\bf Fluid Out}','TexMode','on')
  Bootstrap Reservoir2 : Subsystem  mask(Fluid Reservoir){res_vol=.25, High_Pres_Area=.05, Low_Pres_Area=0, pres_loss=1, T_init=300, P_init=1500, mass_init=30}
      mask prompts: res_vol "Resevoir Volume [m³]"; High_Pres_Area "High Pressure Piston Area"; Low_Pres_Area "Low Pressure Piston Area"; pres_loss "Air Pressure Losses [%]"; T_init "Initial Fluid Temp [K]"; P_init "Initial Air Pressure [kPa]"; mass_init "Initial Fluid Mass [kg]"
      mask help:
      | The fluid reservoir serves as a tank for storing excess hydraulic fluid.
      | The reservoir is fed by returning hydraulic fluid and feeds the engine driven pump.
      | Currently the fluid reservoir tracks the time dependent mass and temperature of the hydraulic fluid in the tank.
      |
      | Block Inputs
      | #1: Bleed air properties (Bus signal)
      | #2: Bypass return from bypass valve
      | #3: Mass flow rate pumped out by hydraulic pump
      | #4: Mass flow rate returned from actuators
      |
      | Block Outputs
      | #1: Bleed air demanded to maintain pressurization
      | #2: Hydraulic fluid properties in the reservoir
      mask init:
      | load AirProp
      | load HydProp
      mask Help: eval('open(''FluidReservoir_help.html'')');
      mask Display:
      | image(imread('hyd_res.png'))
      | 
      | port_label('input',1,'{\bf High Piston Pressure}','TexMode','on')
      | port_label('input',2,'{\bf Bypass Return}','TexMode','on')
      | port_label('input',3,'{\bf m_d_o_t Out}','TexMode','on')
      | port_label('input',4,'{\bf m_d_o_t Return}','TexMode','on')
      | 
      | 
      | port_label('output',1,'{\bf Fluid Out}','TexMode','on')
  Bus Selector1 : BusSelector  OutputSignals=signal1.DC_Voltage_270
  Bus Selector{4..6,8..11,14,16..17} (10 alike) : BusSelector  OutputSignals=mdot_kgps
  Bus Selector12 : BusSelector  OutputSignals=pres_kPa,mdot_kgps
  Bus Selector15 : BusSelector  OutputSignals=Mssn_phase
  Bus Selector3 : BusSelector  OutputSignals=signal1
  Bus Selector7 : BusSelector  OutputSignals=pres_kPa,mdot_kgps
  Bypass Valve1 : PowerFlowLib/Energy & Power Systems/Hydraulic/Bypass Valve
  Bypass Valve2 : PowerFlowLib/Energy & Power Systems/Hydraulic/Bypass Valve
  Constant1 : Constant  Value=Hyd_Pump_Pres
  Constant2 : Constant  Value=Hyd_Pump_Pres
  Constant3 : Constant  Value=DC_Motor_RPM1
  Constant4 : Constant  Value=DC_Motor_RPM2
  DC Speed Servo : Subsystem  AncestorBlock=PowerFlowLib/Energy & Power Systems/Electrical/Machines/DC Speed Servo  mask{Vf=390, Ra=0.05, La=0.9e-3, Rfsh=400, Lfsh=320, Lmsh=1.9, J=1.5}
      mask prompts: Vf "Field voltage (V)"; Ra "Armature resistance (Ohms)"; La "Armature inductance (H)"; Rfsh "Shunt field resistance (Ohms)"; Lfsh "Shunt field inductance (H)"; Lmsh "Mutual inductance (H)"; J "Rotor moment of inertia (Kgm^2)"
  DC Speed Servo1 : Subsystem  AncestorBlock=PowerFlowLib/Energy & Power Systems/Electrical/Machines/DC Speed Servo  mask{Vf=390, Ra=0.05, La=0.9e-3, Rfsh=400, Lfsh=320, Lmsh=1.9, J=1.5}
      mask prompts: Vf "Field voltage (V)"; Ra "Armature resistance (Ohms)"; La "Armature inductance (H)"; Rfsh "Shunt field resistance (Ohms)"; Lfsh "Shunt field inductance (H)"; Lmsh "Mutual inductance (H)"; J "Rotor moment of inertia (Kgm^2)"
  Electric Driven Pump : PowerFlowLib/Energy & Power Systems/Hydraulic/Engine Driven Pump  RPM=3750  disp=39  eta_mech=95  eta_v=85  nom_T=40  nom_w=393  nom_delP=20684
  Electric Driven Pump1 : PowerFlowLib/Energy & Power Systems/Hydraulic/Engine Driven Pump  RPM=3750  disp=39  eta_mech=95  eta_v=85  nom_T=40  nom_w=393  nom_delP=20684
  Hydraulic Load1 : PowerFlowLib/Energy & Power Systems/Hydraulic/Hydraulic Load  fileslct=off  filename=HydraulicLoad.mat  filedir=C:\Users\mwillms4\Dropbox\School\Graduate\Research\PowerFlow Development\PowerFlow Summer 2013\PropertyTables\HydraulicLoad.mat  var_struct=HydraulicLoad  h_load=B_737 - rudder
  Hydraulic Load10 : PowerFlowLib/Energy & Power Systems/Hydraulic/Hydraulic Load  fileslct=off  filename=HydraulicLoad.mat  filedir=C:\Users\mwillms4\Dropbox\School\Graduate\Research\PowerFlow Development\PowerFlow Summer 2013\PropertyTables\HydraulicLoad.mat  var_struct=HydraulicLoad  h_load=B_737 - thrust_rev
  Hydraulic Load2 : PowerFlowLib/Energy & Power Systems/Hydraulic/Hydraulic Load  fileslct=off  filename=HydraulicLoad.mat  filedir=C:\Users\mwillms4\Dropbox\School\Graduate\Research\PowerFlow Development\PowerFlow Summer 2013\PropertyTables\HydraulicLoad.mat  var_struct=HydraulicLoad  h_load=B_737 - ailerons
  Hydraulic Load3 : PowerFlowLib/Energy & Power Systems/Hydraulic/Hydraulic Load  fileslct=off  filename=HydraulicLoad.mat  filedir=C:\Users\mwillms4\Dropbox\School\Graduate\Research\PowerFlow Development\PowerFlow Summer 2013\PropertyTables\HydraulicLoad.mat  var_struct=HydraulicLoad  h_load=B_737 - elevator
  Hydraulic Load4 : PowerFlowLib/Energy & Power Systems/Hydraulic/Hydraulic Load  fileslct=off  filename=HydraulicLoad.mat  filedir=C:\Users\mwillms4\Dropbox\School\Graduate\Research\PowerFlow Development\PowerFlow Summer 2013\PropertyTables\HydraulicLoad.mat  var_struct=HydraulicLoad  h_load=B_737 - landing_gear
  Hydraulic Load5 : PowerFlowLib/Energy & Power Systems/Hydraulic/Hydraulic Load  fileslct=off  filename=HydraulicLoad.mat  filedir=C:\Users\mwillms4\Dropbox\School\Graduate\Research\PowerFlow Development\PowerFlow Summer 2013\PropertyTables\HydraulicLoad.mat  var_struct=HydraulicLoad  h_load=B_737 - rudder
  Hydraulic Load6 : PowerFlowLib/Energy & Power Systems/Hydraulic/Hydraulic Load  fileslct=off  filename=HydraulicLoad.mat  filedir=C:\Users\mwillms4\Dropbox\School\Graduate\Research\PowerFlow Development\PowerFlow Summer 2013\PropertyTables\HydraulicLoad.mat  var_struct=HydraulicLoad  h_load=B_737 - ailerons
  Hydraulic Load7 : PowerFlowLib/Energy & Power Systems/Hydraulic/Hydraulic Load  fileslct=off  filename=HydraulicLoad.mat  filedir=C:\Users\mwillms4\Dropbox\School\Graduate\Research\PowerFlow Development\PowerFlow Summer 2013\PropertyTables\HydraulicLoad.mat  var_struct=HydraulicLoad  h_load=B_737 - elevator
  Hydraulic Load8 : PowerFlowLib/Energy & Power Systems/Hydraulic/Hydraulic Load  fileslct=off  filename=HydraulicLoad.mat  filedir=C:\Users\mwillms4\Dropbox\School\Graduate\Research\PowerFlow Development\PowerFlow Summer 2013\PropertyTables\HydraulicLoad.mat  var_struct=HydraulicLoad  h_load=B_737 - landing_gear
  Hydraulic Load9 : PowerFlowLib/Energy & Power Systems/Hydraulic/Hydraulic Load  fileslct=off  filename=HydraulicLoad.mat  filedir=C:\Users\mwillms4\Dropbox\School\Graduate\Research\PowerFlow Development\PowerFlow Summer 2013\PropertyTables\HydraulicLoad.mat  var_struct=HydraulicLoad  h_load=B_737 - thrust_rev
  Memory : Memory
  Memory1 : Memory
  Mux{1..4} (4 alike) : Mux  Inputs=5
  Scope : Scope
  Scope1 : Scope
      settings: SaveName=ScopeData2
  Sinks : Subsystem
  Terminator : Terminator
  Terminator1 : Terminator
  Terminator2 : Terminator
  To Workspace1 : ToWorkspace  VariableName=hydload5  SampleTime=10  SaveFormat=Structure With Time
  To Workspace2 : ToWorkspace  VariableName=hydload6  SampleTime=10  SaveFormat=Structure With Time
  wires:
  Bus Selector15/1 -> [flight_phase]  "<Mssn_phase>"
  Mission/1 -> Bus Selector15/1
  DC Speed Servo/1(w_m) -> Electric Driven Pump/2, [DC_Motor_RPM3]
  Bus Selector1/1 -> DC Speed Servo/3(Voltage)  "<DC_Voltage_270>"
  Hydraulic Load5/1 -> Bus Selector5/1
  Bypass Valve2/1 -> Hydraulic Load9/1, Hydraulic Load8/1, Hydraulic Load7/1, Hydraulic Load6/1, Hydraulic Load5/1
  Hydraulic Load6/2 -> Mux3/2
  Hydraulic Load7/2 -> Mux3/3
  Hydraulic Load6/1 -> Bus Selector8/1
  Hydraulic Load7/1 -> Bus Selector9/1
  Bus Selector8/1 -> Mux2/2  "<mdot_kgps>"
  Bus Selector5/1 -> Mux2/1  "<mdot_kgps>"
  Bus Selector9/1 -> Mux2/3  "<mdot_kgps>"
  Mux2/1 -> [return_sysA3]
  [flight_phase] -> Hydraulic Load9/2, Hydraulic Load8/2, Hydraulic Load5/2, Hydraulic Load6/2, Hydraulic Load7/2
  Hydraulic Load8/1 -> Bus Selector10/1
  Hydraulic Load9/1 -> Bus Selector11/1
  Hydraulic Load9/2 -> Mux3/5
  Hydraulic Load8/2 -> Mux3/4
  Bus Selector10/1 -> Mux2/4  "<mdot_kgps>"
  Bus Selector11/1 -> Mux2/5  "<mdot_kgps>"
  Hydraulic Load5/2 -> Mux3/1
  Mux3/1 -> To Workspace1/1
  Electric Driven Pump/1 -> Bus Selector12/1, Bypass Valve2/1
  [return_sysA3] -> Bypass Valve2/2
  Constant1/1 -> Electric Driven Pump/3
  Electric Driven Pump/2 -> [Electric_Pump_Torque_Load3]
  [Electric_Pump_Torque_Load3] -> DC Speed Servo/1(T_load (Nm))
  Bypass Valve2/2 -> Memory/1
  [bypass_elec_pump5] -> Bootstrap Reservoir2/2(Bypass Return)
  Bootstrap Reservoir2/1(Fluid Conditions) -> Electric Driven Pump/1
  Constant3/1 -> DC Speed Servo/2(Speed_ref (RPM))
  Bus Selector12/1 -> Scope/1, [Hyd_Fluid_High_Pres5]  "<pres_kPa>"
  Bus Selector12/2 -> [mdot_out5]  "<mdot_kgps>"
  DC Speed Servo/4(Ploss) -> [Motor_PLoss1]
  [Motor_PLoss1] -> Sinks/1("Motor PLoss 1 ")
  DC Speed Servo/2(i_load) -> [Hyd_DC_Motor_Load1]
  [Hyd_DC_Motor_Load1] -> Sinks/3(Motor Current Load 1)
  [return_sysA3] -> Bootstrap Reservoir2/4(Return)
  [mdot_out5] -> Bootstrap Reservoir2/3(mdot_out)
  [Hyd_Fluid_High_Pres5] -> Bootstrap Reservoir2/1(Piston Pressure)
  DC Speed Servo1/1(w_m) -> Electric Driven Pump1/2, [DC_Motor_RPM4]
  [Elec] -> Bus Selector3/1
  Bus Selector3/1 -> DC Speed Servo1/3(Voltage)  "<signal1>"
  Hydraulic Load1/1 -> Bus Selector14/1
  Bypass Valve1/1 -> Hydraulic Load10/1, Hydraulic Load4/1, Hydraulic Load3/1, Hydraulic Load2/1, Hydraulic Load1/1
  Hydraulic Load2/2 -> Mux4/2
  Hydraulic Load3/2 -> Mux4/3
  Hydraulic Load2/1 -> Bus Selector16/1
  Hydraulic Load3/1 -> Bus Selector17/1
  Bus Selector16/1 -> Mux1/2  "<mdot_kgps>"
  Bus Selector14/1 -> Mux1/1  "<mdot_kgps>"
  Bus Selector17/1 -> Mux1/3  "<mdot_kgps>"
  Mux1/1 -> [return_sysB3]
  [flight_phase] -> Hydraulic Load10/2, Hydraulic Load4/2, Hydraulic Load1/2, Hydraulic Load2/2, Hydraulic Load3/2
  Hydraulic Load4/1 -> Bus Selector4/1
  Hydraulic Load10/1 -> Bus Selector6/1
  Hydraulic Load10/2 -> Mux4/5
  Hydraulic Load4/2 -> Mux4/4
  Bus Selector4/1 -> Mux1/4  "<mdot_kgps>"
  Bus Selector6/1 -> Mux1/5  "<mdot_kgps>"
  Hydraulic Load1/2 -> Mux4/1
  Mux4/1 -> To Workspace2/1
  Electric Driven Pump1/1 -> Bus Selector7/1, Bypass Valve1/1
  [return_sysB3] -> Bypass Valve1/2
  Constant2/1 -> Electric Driven Pump1/3
  Electric Driven Pump1/2 -> [Electric_Pump_Torque_Load]
  [Electric_Pump_Torque_Load] -> DC Speed Servo1/1(T_load (Nm))
  Bypass Valve1/2 -> Memory1/1
  [bypass_elec_pump6] -> Bootstrap Reservoir1/2(Bypass Return)
  Bootstrap Reservoir1/1(Fluid Conditions) -> Electric Driven Pump1/1
  Constant4/1 -> DC Speed Servo1/2(Speed_ref (RPM))
  Bus Selector7/1 -> Scope1/1, [Hyd_Fluid_High_Pres6]  "<pres_kPa>"
  Bus Selector7/2 -> [mdot_out6]  "<mdot_kgps>"
  DC Speed Servo1/4(Ploss) -> [Motor_PLoss2]
  DC Speed Servo1/2(i_load) -> [Hyd_DC_Motor_Load2]
  [return_sysB3] -> Bootstrap Reservoir1/4(Return)
  [mdot_out6] -> Bootstrap Reservoir1/3(mdot_out)
  [Hyd_Fluid_High_Pres6] -> Bootstrap Reservoir1/1(Piston Pressure)
  [Motor_PLoss2] -> Sinks/2(Motor PLoss 2)
  [Hyd_DC_Motor_Load2] -> Sinks/4(Motor Current Load 2)
  [Elec] -> Bus Selector1/1
  Elec/1 -> [Elec]
  Sinks/1(Out1) -> Terminator/1
  DC Speed Servo1/3(T_em) -> Terminator2/1
  DC Speed Servo/3(T_em) -> Terminator1/1
  Memory/1 -> [bypass_elec_pump5]
  Memory1/1 -> [bypass_elec_pump6]
